simulink model "obs_sys"  (Simulink 8.6)
settings: Solver=ode45  StartTime=0.0  StopTime=5  MaxStep=0.001  RelTol=1e-3
settings Model: Creator=Thomas Chmielewski  LastModifiedBy=DR_C
settings OptimizationCC: InitFltsAndDblsToZero=on
settings DebuggingCC: SaveWithParameterizedLinksMsg=none  SignalResolutionControl=TryResolveAllWithWarning  SolverPrmCheckMsg=none  MultiTaskDSMMsg=warning  MultiTaskCondExecSysMsg=none  FcnCallInpInsideContextMsg=UseLocalSettings
settings HardwareCC: TargetUnknown=on
settings GRTTargetCC: TargetFcnLib=ansi_tfl_tmw.mat  CompOptLevelCompliant=off

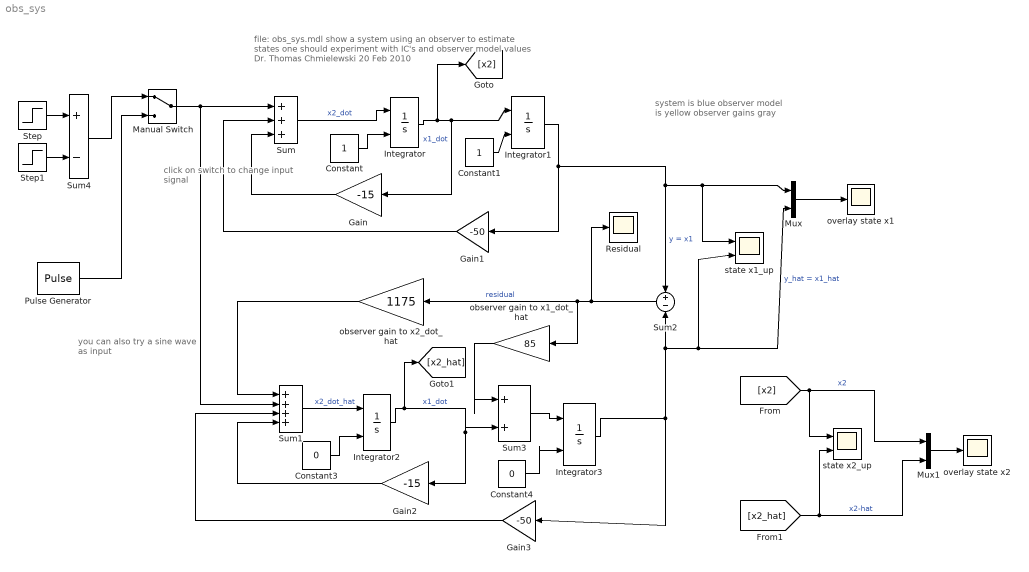
== system obs_sys ==
  note: system is blue
      | observer model is yellow
      | observer gains gray
  note: file:  obs_sys.mdl
      | show a system using an observer to estimate states
      | one should experiment with IC's and observer model values
      | Dr. Thomas Chmielewski
      | 20 Feb 2010
  note: click on switch
      | to change
      | input signal
  note: you can also try
      | a sine wave as input
  Constant : Constant
  Constant1 : Constant
  Constant3 : Constant  Value=0
  Constant4 : Constant  Value=0
  Gain : Gain  Gain=-15
  Gain1 : Gain  Gain=-50
  Gain2 : Gain  Gain=-15
  Gain3 : Gain  Gain=-50
  Integrator : Integrator  InitialConditionSource=external  InitialCondition=1
  Integrator1 : Integrator  InitialConditionSource=external  InitialCondition=10
  Integrator2 : Integrator  InitialConditionSource=external
  Integrator3 : Integrator  InitialConditionSource=external
  Manual Switch : ManualSwitch
  Mux : Mux  Inputs=2
  Mux1 : Mux  Inputs=2
  Pulse Generator : DiscretePulseGenerator  PulseType=Time based  Period=1  PulseWidth=25
  Residual : Scope
  Step : Step  SampleTime=0
  Step1 : Step  Time=3  SampleTime=0
  Sum : Sum  Inputs=+++
  Sum1 : Sum  Inputs=++++
  Sum2 : Sum  Inputs=+-
  Sum3 : Sum  Inputs=|++
  Sum4 : Sum  Inputs=+-
  observer gain to x1_dot_hat : Gain  Gain=85
  observer gain to x2_dot_hat : Gain  Gain=1175
  overlay state x1 : Scope
  overlay state x2 : Scope
  state x1_up : Scope  NumInputPorts=2
  state x2_up : Scope  NumInputPorts=2
  wires:
  Integrator/1 -> Integrator1/1, Gain/1, [x2]  "x1_dot"
  Sum/1 -> Integrator/1  "x2_dot"
  Integrator1/1 -> Gain1/1, Sum2/1, Mux/1, state x1_up/1  "y = x1"
  Gain/1 -> Sum/3
  Gain1/1 -> Sum/2
  Integrator2/1 -> Sum3/2, Gain2/1, [x2_hat]  "x1_dot"
  Sum1/1 -> Integrator2/1  "x2_dot_hat"
  Integrator3/1 -> Gain3/1, Sum2/2, Mux/2, state x1_up/2  "y_hat = x1_hat"
  Gain2/1 -> Sum1/4
  Gain3/1 -> Sum1/3
  observer gain to x2_dot_hat/1 -> Sum1/1
  Sum3/1 -> Integrator3/1
  observer gain to x1_dot_hat/1 -> Sum3/1
  Sum2/1 -> observer gain to x2_dot_hat/1, observer gain to x1_dot_hat/1, Residual/1  "residual"
  Mux/1 -> overlay state x1/1
  Mux1/1 -> overlay state x2/1
  [x2] -> Mux1/1, state x2_up/1  "x2"
  [x2_hat] -> Mux1/2, state x2_up/2  "x2-hat"
  Constant/1 -> Integrator/2
  Constant1/1 -> Integrator1/2
  Step/1 -> Sum4/1
  Step1/1 -> Sum4/2
  Pulse Generator/1 -> Manual Switch/2
  Constant4/1 -> Integrator3/2
  Constant3/1 -> Integrator2/2
  Manual Switch/1 -> Sum/1, Sum1/2
  Sum4/1 -> Manual Switch/1
